simulink model "PresaDepredador_control"  (R2020a)
settings: Solver=VariableStepAuto  StartTime=0.0  StopTime=Time  RelTol=1e-3
undefined symbols (not defined in the file): alpha, Amplitude, beta, D0, delta, Frequency, gamma, K, P0
settings Model: Creator=curie  LastModifiedBy=curie
settings DataIOCC: ReturnWorkspaceOutputs=off

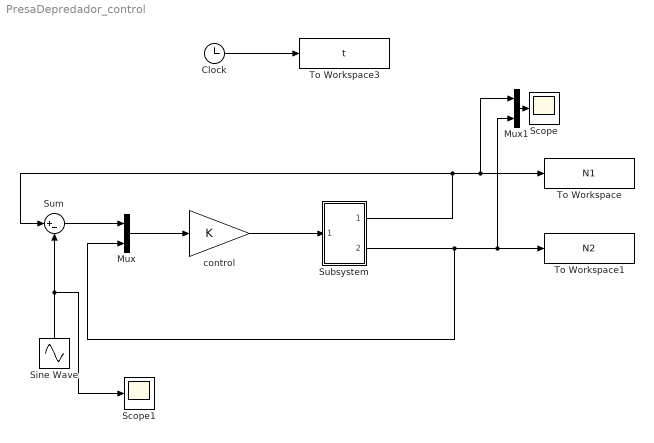
== system PresaDepredador_control ==
  Clock : Clock
  Mux : Mux  Inputs=2
  Mux1 : Mux  Inputs=2
  Scope : Scope
  Scope1 : Scope
  Sine Wave : Sin  Amplitude=Amplitude  Bias=u  Frequency=Frequency  SampleTime=0
  Subsystem : Subsystem
  Sum : Sum  Inputs=|+-
  To Workspace : ToWorkspace  VariableName=N1  SampleTime=-1
  To Workspace1 : ToWorkspace  VariableName=N2  SampleTime=-1
  To Workspace3 : ToWorkspace  VariableName=t  SampleTime=-1
  control : Gain  Gain=K
  wires:
  Clock/1 -> To Workspace3/1
  Sine Wave/1 -> Scope1/1, Sum/2
  Mux/1 -> control/1
  control/1 -> Subsystem/1(In1)
  Subsystem/1(Out1) -> Sum/1, Mux1/1, To Workspace/1
  Subsystem/2(Out2) -> Mux1/2, To Workspace1/1, Mux/2
  Mux1/1 -> Scope/1
  Sum/1 -> Mux/1

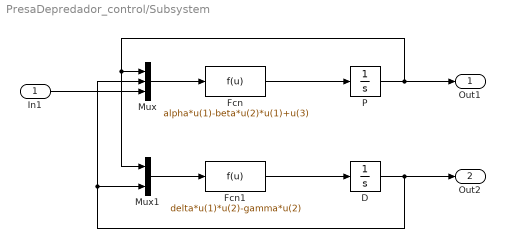
== system PresaDepredador_control/Subsystem ==
  In1 : Inport
  D : Integrator  InitialCondition=D0  LimitOutput=on  LowerSaturationLimit=0  ZeroCross=off
  Fcn : Fcn  Expr=alpha*u(1)-beta*u(2)*u(1)+u(3)
  Fcn1 : Fcn  Expr=delta*u(1)*u(2)-gamma*u(2)
  Mux : Mux  Inputs=3
  Mux1 : Mux  Inputs=2
  P : Integrator  InitialCondition=P0  LimitOutput=on  LowerSaturationLimit=0  ZeroCross=off
  Out1 : Outport
  Out2 : Outport  Port=2
  wires:
  Mux/1 -> Fcn/1
  Mux1/1 -> Fcn1/1
  Fcn/1 -> P/1
  D/1 -> Out2/1, Mux/2, Mux1/2
  P/1 -> Out1/1, Mux1/1, Mux/1
  In1/1 -> Mux/3
  Fcn1/1 -> D/1
